simulink model "light_"  (R2021a)
settings: Solver=FixedStepDiscrete  StartTime=0.0  StopTime=20  FixedStep=0.5  RelTol=1e-3
CloseFcn:
  | clear all
  | try
  | rmdir slprj\ s
  | catch
  | end
  | try
  | folder_name = [bdroot '*'];
  | rmdir(folder_name,'s')
  | catch
  | end
  | try
  | file_temp_name = [bdroot '.slxc'];
  | delete(file_temp_name)
  | %%delete *.mexw64
  | catch
  | end
  | clear folder_name file_temp_name
settings Model: Creator=jetson  LastModifiedBy=jetson
settings DataIOCC: SaveOutput=off  SignalLogging=off  DSMLogging=off  SaveTime=off  ReturnWorkspaceOutputs=off
settings OptimizationCC: DefaultParameterBehavior=Inlined  EnhancedBackFolding=on  PassReuseOutputArgsAs=Individual arguments  ZeroExternalMemoryAtStartup=off  ZeroInternalMemoryAtStartup=off  OptimizeBlockOrder=speed  DifferentSizesBufferReuse=on  OptimizationCustomize=off  EfficientTunableParamExpr=on
settings DebuggingCC: ParameterTunabilityLossMsg=error
settings SFSimCC: MATLABDynamicMemAlloc=off
settings RTWCC: SystemTargetFile=ert.tlc  GenCodeOnly=on  TemplateMakefile=ert_default_tmf  GenerateReport=on  RTWUseSimCustomCode=on  IncludeHyperlinkInReport=on  LaunchReport=on  GenerateTraceInfo=on
settings CodeAppCC: ForceParamTrailComments=on  IgnoreCustomStorageClasses=off  OperatorAnnotations=on  SimulinkDataObjDesc=on  SFDataObjDesc=on  InsertBlockDesc=on
settings ERTTargetCC: TargetLangStandard=C99 (ISO)  GenerateSampleERTMain=on  InlinedParameterPlacement=NonHierarchical  ERTCustomFileTemplate=example_file_process.tlc

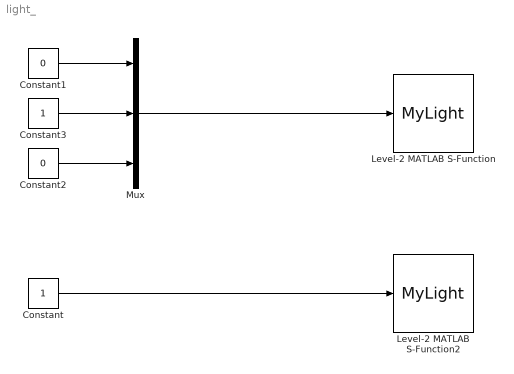
== system light_ ==
  Constant : Constant
  Constant1 : Constant  Value=0
  Constant2 : Constant  Value=0
  Constant3 : Constant
  Level-2 MATLAB S-Function : M-S-Function  FunctionName=MyLight
      mask Display:
      | t = 0: .05:2*pi;
      | x= sin(t)/2 + 0.5;
      | y = cos(t)/2 + 0.5;
      | patch(x, y,[0 1 0])
  Level-2 MATLAB S-Function2 : M-S-Function  FunctionName=MyLight
      mask Display:
      | color('red')
      | r = linspace(0,1, 10000);
      | t = linspace(0, 500*pi, 10000);
      | x = r.*sin(t)/2 + 0.5;
      | y = r.*cos(t)/2 + 0.5;
      | plot(x, y)
  Mux : Mux  Inputs=3
  wires:
  Constant2/1 -> Mux/3
  Mux/1 -> Level-2 MATLAB S-Function/1
  Constant/1 -> Level-2 MATLAB S-Function2/1
  Constant1/1 -> Mux/1
  Constant3/1 -> Mux/2
